simulink model "AMR_MotorControlUnit_24a"  (R2024a)
settings: configuration reference "SharedConfig" (kept outside this file)
undefined symbols (not defined in the file): min_motor_rpm, mobotic_mechanical_offset
settings Model: DataDictionary=configuration_dictionary.sldd  Creator=matlab.cut  LastModifiedBy=matlab.cut
settings ConfigSetRef: SourceName=SharedConfig

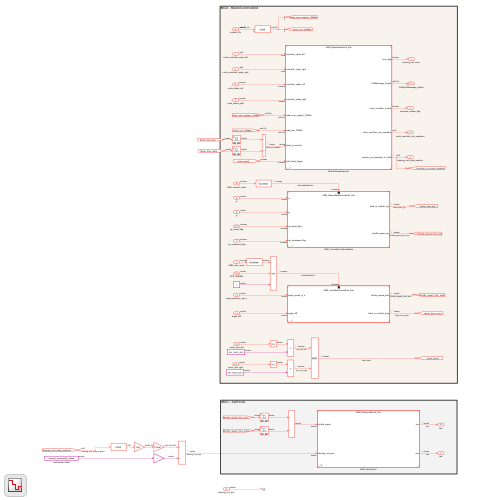
[thumbnail: Simulink's stored preview of the top-level diagram]
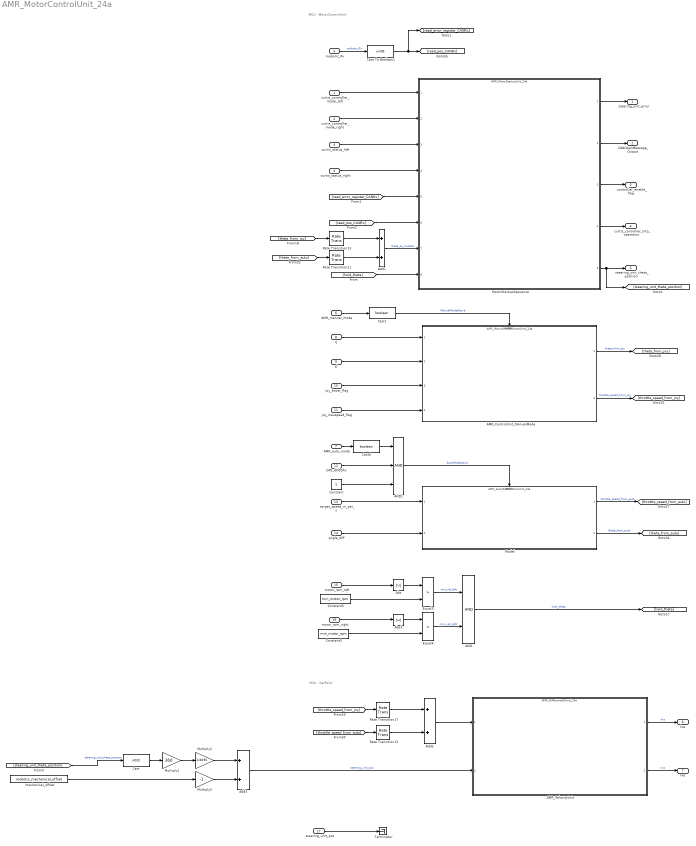
== system AMR_MotorControlUnit_24a ==
  note: MCU - MotorControlUnit
  note: MCU - SetPoint
  curtis_controller_mode_left : Inport
  curtis_controller_mode_right : Inport  Port=2
  curtis_status_left : Inport  Port=3
  curtis_status_right : Inport  Port=4
  mobotic_Rx : Inport  Port=5
  AMR_manual_mode : Inport  Port=6  OutDataTypeStr=boolean
  AMR_auto_mode : Inport  Port=7  OutDataTypeStr=boolean
  xj : Inport  Port=8
  yj : Inport  Port=9
  joy_boost_flag : Inport  Port=10
  joy_maxspeed_flag : Inport  Port=11
  GPS_GNSSfix : Inport  Port=12
  target_speed_m_per_s : Inport  Port=13
  angle_diff : Inport  Port=14
  motor_rpm_left : Inport  Port=15
  motor_rpm_right : Inport  Port=16
  steering_unit_pos : Inport  Port=17
  AMR_ControlUnit_ManualMode : ModelReference  ModelNameDialog=AMR_ManualModeControlUnit_24a.slx  SimulationMode=Normal  ModelReferenceVersion=2.12  EnablePortName=Enable  EnablePortStatesWhenEnabling=held
  AMR_VelocityUnit : ModelReference  ModelNameDialog=AMR_DifferentialDrive_24a  SimulationMode=Normal  ModelReferenceVersion=2.16
  AND : Logic  AllPortsSameDT=off  OutDataTypeStr=boolean
  AND1 : Logic  Inputs=3  AllPortsSameDT=off  OutDataTypeStr=boolean
  Abs : Abs  SaturateOnIntegerOverflow=off
  Abs3 : Abs  SaturateOnIntegerOverflow=off
  Add1 : Sum
  Add2 : Sum
  Add3 : Sum
  Cast : DataTypeConversion  OutDataTypeStr=int32  SaturateOnIntegerOverflow=off  RndMeth=Floor
  Cast To Boolean1 : DataTypeConversion  OutDataTypeStr=uint8  SaturateOnIntegerOverflow=off  RndMeth=Floor
  Cast1 : DataTypeConversion  OutDataTypeStr=boolean  SaturateOnIntegerOverflow=off  RndMeth=Floor
  Cast6 : DataTypeConversion  OutDataTypeStr=boolean  SaturateOnIntegerOverflow=off  RndMeth=Floor
  Constant : Constant
  Constant3 : Constant  Value=min_motor_rpm
  Constant5 : Constant  Value=min_motor_rpm
  Equal3 : RelationalOperator  Operator=>  OutDataTypeStr=boolean  RndMeth=Simplest  InputSameDT=off
  Equal4 : RelationalOperator  Operator=>  OutDataTypeStr=boolean  RndMeth=Simplest  InputSameDT=off
  Model : ModelReference  ModelNameDialog=AMR_AutoModeControlUnit_24a  SimulationMode=Normal  ModelReferenceVersion=2.18  EnablePortName=Enable  EnablePortStatesWhenEnabling=held
  MotorStartupSequence : ModelReference  ModelNameDialog=AMR_MotorStartupUnit_24a.slx  SimulationMode=Normal  ModelReferenceVersion=2.44
  Multiply1 : Gain  Gain=360
  Multiply2 : Gain  Gain=1/4096
  Multiply3 : Gain  Gain=-1
  Rate Transition{11..13,17} (4 alike) : RateTransition
  Terminator : Terminator
  mechanical_offset : Constant  Value=mobotic_mechanical_offset
  steering_unit_error : Outport
  CANOpenMessage_Output : Outport  Port=2
  controller_enable_flag : Outport  Port=3
  curtis_controller_into_operation : Outport  Port=4
  steering_unit_theta_position : Outport  Port=5
  lws : Outport  Port=6
  rws : Outport  Port=7
  wires:
  Cast1/1 -> AMR_ControlUnit_ManualMode/Enable  "ManualModeActive"
  curtis_status_right/1 -> MotorStartupSequence/4
  xj/1 -> AMR_ControlUnit_ManualMode/1
  curtis_controller_mode_right/1 -> MotorStartupSequence/2
  curtis_controller_mode_left/1 -> MotorStartupSequence/1
  joy_maxspeed_flag/1 -> AMR_ControlUnit_ManualMode/4
  AMR_ControlUnit_ManualMode/2 -> [throttle_speed_from_joy]  "throttle_speed_from_joy"
  [theta_from_auto] -> Rate Transition11/1
  AMR_ControlUnit_ManualMode/1 -> [theta_from_joy]  "theta_from_joy"
  AMR_VelocityUnit/2 -> rws/1  "rws"
  yj/1 -> AMR_ControlUnit_ManualMode/2
  [hold_theta] -> MotorStartupSequence/8
  Add1/1 -> MotorStartupSequence/7  "theta_to_mobotic"
  [throttle_speed_from_auto] -> Rate Transition12/1
  AMR_VelocityUnit/1 -> lws/1  "lws"
  Add2/1 -> AMR_VelocityUnit/1
  [theta_from_joy] -> Rate Transition13/1
  curtis_status_left/1 -> MotorStartupSequence/3
  Rate Transition11/1 -> Add1/2
  Constant/1 -> AND1/3
  GPS_GNSSfix/1 -> AND1/2
  AMR_auto_mode/1 -> Cast6/1
  target_speed_m_per_s/1 -> Model/1
  [throttle_speed_from_joy] -> Rate Transition17/1
  joy_boost_flag/1 -> AMR_ControlUnit_ManualMode/3
  Rate Transition12/1 -> Add2/2
  AND1/1 -> Model/Enable  "AutoModeActive"
  Rate Transition17/1 -> Add2/1
  Model/1 -> [throttle_speed_from_auto]  "throttle_speed_from_auto"
  Model/2 -> [theta_from_auto]  "theta_from_auto"
  Rate Transition13/1 -> Add1/1
  AMR_manual_mode/1 -> Cast1/1
  motor_rpm_right/1 -> Abs3/1
  Abs3/1 -> Equal4/1
  Equal3/1 -> AND/1  "min_vel_left"
  Abs/1 -> Equal3/1
  motor_rpm_left/1 -> Abs/1
  Equal4/1 -> AND/2  "min_vel_right"
  Constant3/1 -> Equal4/2
  Constant5/1 -> Equal3/2
  AND/1 -> [hold_theta]  "hold_theta"
  Cast6/1 -> AND1/1
  MotorStartupSequence/5 -> [steering_unit_theta_position], steering_unit_theta_position/1
  angle_diff/1 -> Model/2
  Cast To Boolean1/1 -> [read_pos_CANRx], [read_error_register_CANRx]
  mobotic_Rx/1 -> Cast To Boolean1/1  "mobotic_Rx"
  [read_error_register_CANRx] -> MotorStartupSequence/5
  [read_pos_CANRx] -> MotorStartupSequence/6
  MotorStartupSequence/1 -> steering_unit_error/1
  MotorStartupSequence/2 -> CANOpenMessage_Output/1
  MotorStartupSequence/3 -> controller_enable_flag/1
  MotorStartupSequence/4 -> curtis_controller_into_operation/1
  mechanical_offset/1 -> Multiply3/1
  [steering_unit_theta_position] -> Cast/1  "steering_unit_theta_position"
  Multiply1/1 -> Multiply2/1
  Multiply3/1 -> Add3/2
  Multiply2/1 -> Add3/1
  Cast/1 -> Multiply1/1
  Add3/1 -> AMR_VelocityUnit/2  "steering_unit_pos"
  steering_unit_pos/1 -> Terminator/1
